simulink model "FDIA_TRAINING_39_1"  (R2021a)
settings: Solver=ode23tb  StartTime=0.0  StopTime=27  MaxStep=1/60  RelTol=1e-2  AbsTol=1e-1  EnableMultiTasking=on
PreLoadFcn:
  | NE39bus_data;
  | PSSMODEL=1;
  | LPSS=0;
  | WAPSS=0;
  | WAPSS2=0;
undefined symbols (not defined in the file): AVR_Data, D1, Delta, line, mac_con, MB, Ns, p0, Pn, s
libraries: spsThreePhaseVIMeasurementLib x40, spsThreePhasePISectionLineLib x34, simulink x20, spsGenericPowerSystemStabilizerLib x20, spsThreePhaseTransformerTwoWindingsLib x12, spsSynchronousMachinepuStandardLib x10, spsExcitationSystemLib x10, spsMultiBandPowerSystemStabilizerLib x10, spsSteamTurbineandGovernorLib x10, slpidlib x10, spsLoadFlowBusLib x9, spsThreePhaseDynamicLoadLib x9
(part 1 of 4)
settings Model: Creator=Innocent  LastModifiedBy=suman
settings SolverCC: AutoScaleAbsTol=off  AlgebraicLoopSolver=TrustRegion
settings DataIOCC: SaveFormat=Array  SignalLoggingSaveFormat=ModelDataLogs  SaveOutput=off  SaveTime=off  ReturnWorkspaceOutputs=off
settings OptimizationCC: BlockReduction=off  BooleanDataType=off  ExpressionDepthLimit=2147483647  InitFltsAndDblsToZero=on  LifeSpan=inf
settings DebuggingCC: SaveWithParameterizedLinksMsg=none  UnderspecifiedInitializationDetection=Classic  MergeDetectMultiDrivingBlocksExec=none  SignalResolutionControl=TryResolveAllWithWarning  SolverPrmCheckMsg=warning  MultiTaskDSMMsg=warning  MultiTaskCondExecSysMsg=none  FcnCallInpInsideContextMsg=warning  UnconnectedInputMsg=none  UnconnectedOutputMsg=none  UnconnectedLineMsg=none  StateNameClashWarn=warning  StrictBusMsg=ErrorOnBusTreatedAsVector  SFUnexpectedBacktrackingDiag=warning  SFNoUnconditionalDefaultTransitionDiag=warning  SFExecutionAtInitializationDiag=none  SFMachineParentedDataDiag=warning  ArithmeticOperatorsInVariantConditions=warning
settings HardwareCC: ProdBitPerPointer=32  ProdBitPerSizeT=32  ProdBitPerPtrDiffT=32  ProdLargestAtomicFloat=None  ProdIntDivRoundTo=Undefined  ProdEndianess=Unspecified  ProdWordSize=32  ProdHWDeviceType=32-bit Generic
settings ModelReferenceCC: PropagateSignalLabelsOutOfModel=off
settings SFSimCC: SimUseLocalCustomCode=off  CustomCodeUndefinedFunction=UseInterfaceOnly
settings RTWCC: RTWUseLocalCustomCode=off
settings CodeAppCC: StateflowObjectComments=on
settings GRTTargetCC: TargetFcnLib=ansi_tfl_tmw.mat  TargetLangStandard=C89/C90 (ANSI)  CombineOutputUpdateFcns=off  GRTInterface=on
settings ConfigComp: CovMetricSettings=dw  CovSaveCumulativeToWorkspaceVar=on  CovSaveSingleToWorkspaceVar=on  CovExternalEMLEnable=off
settings SimscapeCC: SimscapeNormalizeSystem=off

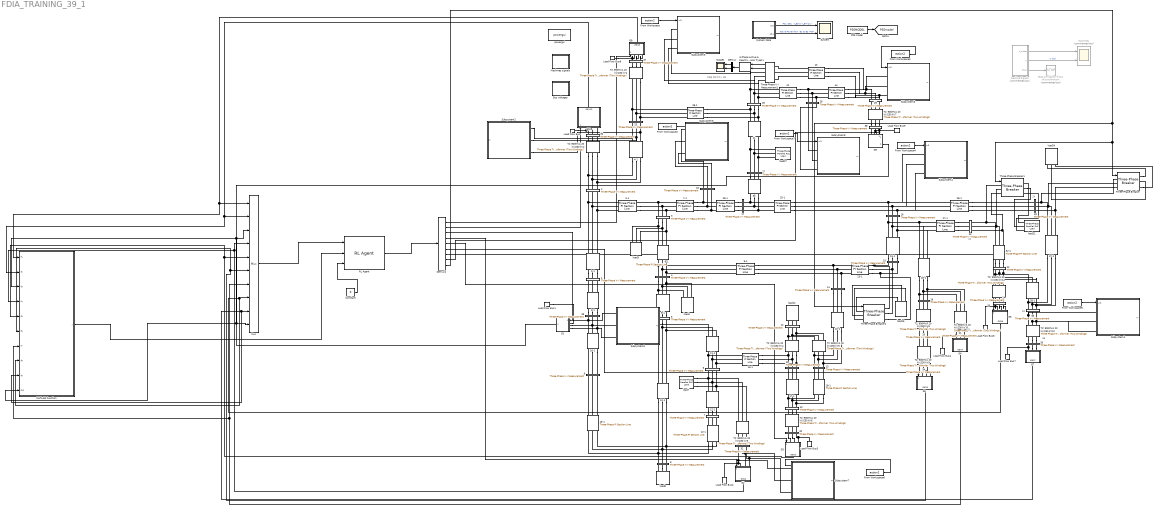
== system FDIA_TRAINING_39_1 ==
  note: 35
  note: 33
  note: 21
  note: 24
  note: 36
  note: P&Q 29 ==> 26
  note: 23
  " 30" : spsThreePhasePISectionLineLib/Three-Phase PI Section Line  LConnTagsString=a|b|c  RConnTagsString=A|B|C  Length=1  Frequency=50  Resistances="[line(30,3)  3*line(30,3)]"  Inductances="[line(30,4)  3*line(30,4)]"  Capacitances="[line(30,5)  line(30,5)/3]"
  1 : spsThreePhaseVIMeasurementLib/Three-Phase V-I Measurement  VoltageMeasurement=phase-to-phase  SetLabelV=on  LabelV=Vabc_1  Vpu=off  VpuLL=on  CurrentMeasurement=no  SetLabelI=on  LabelI=Iabc_B2  Ipu=off  Pbase=100e6  Vbase=Bus(1,2)*1e3  OutputType=Complex  PhasorSimulation=on  PSBequivalent=0
  1-1 : spsThreePhasePISectionLineLib/Three-Phase PI Section Line  LConnTagsString=a|b|c  RConnTagsString=A|B|C  Length=1  Frequency=50  Resistances="[line(1,3)  3*line(1,3)]"  Inductances="[line(1,4)  3*line(1,4)]"  Capacitances="[line(1,5)  line(1,5)/3]"
  10 : spsThreePhaseVIMeasurementLib/Three-Phase V-I Measurement  VoltageMeasurement=phase-to-phase  SetLabelV=on  LabelV=Vabc_10  Vpu=off  VpuLL=on  CurrentMeasurement=no  SetLabelI=on  LabelI=Iabc_B2  Ipu=off  Pbase=100e6  Vbase=Bus(10,2)*1e3  OutputType=Complex  PhasorSimulation=on  PSBequivalent=0
  10-1 : spsThreePhasePISectionLineLib/Three-Phase PI Section Line  LConnTagsString=a|b|c  RConnTagsString=A|B|C  Length=1  Frequency=50  Resistances="[line(10,3)  3*line(10,3)]"  Inductances="[line(10,4)  3*line(10,4)]"  Capacitances="[line(10,5)  line(10,5)/3]"
  11 : spsThreePhaseVIMeasurementLib/Three-Phase V-I Measurement  VoltageMeasurement=phase-to-phase  SetLabelV=on  LabelV=Vabc_11  Vpu=off  VpuLL=on  CurrentMeasurement=no  SetLabelI=on  LabelI=Iabc_B2  Ipu=off  Pbase=100e6  Vbase=Bus(11,2)*1e3  OutputType=Complex  PhasorSimulation=on  PSBequivalent=0
  11-1 : spsThreePhasePISectionLineLib/Three-Phase PI Section Line  LConnTagsString=a|b|c  RConnTagsString=A|B|C  Length=1  Frequency=50  Resistances="[line(11,3)  3*line(11,3)]"  Inductances="[line(11,4)  3*line(11,4)]"  Capacitances="[line(11,5)   line(11,5)/3]"
  12 : spsThreePhaseVIMeasurementLib/Three-Phase V-I Measurement  VoltageMeasurement=phase-to-phase  SetLabelV=on  LabelV=Vabc_12  Vpu=off  VpuLL=on  CurrentMeasurement=no  SetLabelI=on  LabelI=Iabc_B2  Ipu=off  Pbase=100e6  Vbase=Bus(12,2)*1e3  OutputType=Complex  PhasorSimulation=on  PSBequivalent=0
  12-1 : spsThreePhasePISectionLineLib/Three-Phase PI Section Line  LConnTagsString=a|b|c  RConnTagsString=A|B|C  Length=1  Frequency=50  Resistances="[line(12,3)  3*line(12,3)]"  Inductances="[line(12,4)  3*line(12,4)]"  Capacitances="[line(12,5)   line(12,5)/3]"
  13 : spsThreePhaseVIMeasurementLib/Three-Phase V-I Measurement  VoltageMeasurement=phase-to-phase  SetLabelV=on  LabelV=Vabc_13  Vpu=off  VpuLL=on  CurrentMeasurement=no  SetLabelI=on  LabelI=Iabc_B2  Ipu=off  Pbase=100e6  Vbase=Bus(13,2)*1e3  OutputType=Complex  PhasorSimulation=on  PSBequivalent=0
  13-1 : spsThreePhasePISectionLineLib/Three-Phase PI Section Line  LConnTagsString=a|b|c  RConnTagsString=A|B|C  Length=1  Frequency=50  Resistances=[line(13,3) 3*line(13,3)]  Inductances="[line(13,4)  3*line(13,4)]"  Capacitances="[line(13,5)  line(13,5)/3]"
  14 : spsThreePhaseVIMeasurementLib/Three-Phase V-I Measurement  VoltageMeasurement=phase-to-phase  SetLabelV=on  LabelV=Vabc_14  Vpu=off  VpuLL=on  CurrentMeasurement=no  SetLabelI=on  LabelI=Iabc_B2  Ipu=off  Pbase=100e6  Vbase=Bus(14,2)*1e3  OutputType=Complex  PhasorSimulation=on  PSBequivalent=0
  14-1 : spsThreePhasePISectionLineLib/Three-Phase PI Section Line  LConnTagsString=a|b|c  RConnTagsString=A|B|C  Length=1  Frequency=50  Resistances=[ line(14,3) 3*line(14,3)]  Inductances="[ line(14,4)  3*line(14,4)]"  Capacitances="[line(14,5)   line(14,5)/3]"
  15 : spsThreePhaseVIMeasurementLib/Three-Phase V-I Measurement  VoltageMeasurement=phase-to-phase  SetLabelV=on  LabelV=Vabc_15  Vpu=off  VpuLL=on  CurrentMeasurement=no  SetLabelI=on  LabelI=Iabc_B2  Ipu=off  Pbase=100e6  Vbase=Bus(15,2)*1e3  OutputType=Complex  PhasorSimulation=on  PSBequivalent=0
  15-1 : spsThreePhasePISectionLineLib/Three-Phase PI Section Line  LConnTagsString=a|b|c  RConnTagsString=A|B|C  Length=1  Frequency=50  Resistances="[line(15,3)  3*line(15,3)]"  Inductances="[line(15,4)  3*line(15,4)]"  Capacitances="[line(15,5)   line(15,5)/5]"
  16 : spsThreePhaseVIMeasurementLib/Three-Phase V-I Measurement  VoltageMeasurement=phase-to-phase  SetLabelV=on  LabelV=Vabc_16  Vpu=off  VpuLL=on  CurrentMeasurement=no  SetLabelI=on  LabelI=Iabc_B2  Ipu=off  Pbase=100e6  Vbase=Bus(16,2)*1e3  OutputType=Complex  PhasorSimulation=on  PSBequivalent=0
  16-1 : spsThreePhasePISectionLineLib/Three-Phase PI Section Line  LConnTagsString=a|b|c  RConnTagsString=A|B|C  Length=1  Frequency=50  Resistances="[line(8,3)  3*line(8,3)]"  Inductances="[line(8,4)  3*line(8,4)]"  Capacitances="[line(8,5)   line(8,5)/3]"
  17 : spsThreePhaseVIMeasurementLib/Three-Phase V-I Measurement  VoltageMeasurement=phase-to-phase  SetLabelV=on  LabelV=Vabc_17  Vpu=off  VpuLL=on  CurrentMeasurement=no  SetLabelI=on  LabelI=Iabc_B2  Ipu=off  Pbase=100e6  Vbase=Bus(17,2)*1e3  OutputType=Complex  PhasorSimulation=on  PSBequivalent=0
  17-1 : spsThreePhasePISectionLineLib/Three-Phase PI Section Line  LConnTagsString=a|b|c  RConnTagsString=A|B|C  Length=1  Frequency=50  Resistances="[line(17,3)  3*line(17,3)]"  Inductances="[line(17,4)  3*line(17,4)]"  Capacitances="[line(17,5)   line(17,5)/3]"
  18 : spsThreePhaseVIMeasurementLib/Three-Phase V-I Measurement  VoltageMeasurement=phase-to-phase  SetLabelV=on  LabelV=Vabc_18  Vpu=off  VpuLL=on  CurrentMeasurement=no  SetLabelI=on  LabelI=Iabc_B2  Ipu=off  Pbase=100e6  Vbase=Bus(18,2)*1e3  OutputType=Complex  PhasorSimulation=on  PSBequivalent=0
  18-1 : spsThreePhasePISectionLineLib/Three-Phase PI Section Line  LConnTagsString=a|b|c  RConnTagsString=A|B|C  Length=1  Frequency=50  Resistances="[line(18,3)  3*line(18,3)]"  Inductances="[line(18,4)  3*line(18,4)]"  Capacitances="[line(18,5)   line(18,5)/3]"
  19 : spsThreePhaseVIMeasurementLib/Three-Phase V-I Measurement  VoltageMeasurement=phase-to-phase  SetLabelV=on  LabelV=Vabc_19  Vpu=off  VpuLL=on  CurrentMeasurement=no  SetLabelI=on  LabelI=Iabc_B2  Ipu=off  Pbase=100e6  Vbase=Bus(19,2)*1e3  OutputType=Complex  PhasorSimulation=on  PSBequivalent=0
  2 : spsThreePhaseVIMeasurementLib/Three-Phase V-I Measurement  VoltageMeasurement=phase-to-phase  SetLabelV=on  LabelV=Vabc_2  Vpu=off  VpuLL=on  CurrentMeasurement=no  SetLabelI=on  LabelI=Iabc_B2  Ipu=off  Pbase=100e6  Vbase=Bus(2,2)*1e3  OutputType=Complex  PhasorSimulation=on  PSBequivalent=0
  2-1 : spsThreePhasePISectionLineLib/Three-Phase PI Section Line  LConnTagsString=a|b|c  RConnTagsString=A|B|C  Length=1  Frequency=50  Resistances="[line(2,3)  3*line(2,3)]"  Inductances="[line(2,4)  3*line(2,4)]"  Capacitances="[line(2,5)   line(2,5)/3]"
  20 : spsThreePhaseVIMeasurementLib/Three-Phase V-I Measurement  VoltageMeasurement=phase-to-phase  SetLabelV=on  LabelV=Vabc_20  Vpu=off  VpuLL=on  CurrentMeasurement=no  SetLabelI=on  LabelI=Iabc_B2  Ipu=off  Pbase=100e6  Vbase=Bus(20,2)*1e3  OutputType=Complex  PhasorSimulation=on  PSBequivalent=0
  21 : spsThreePhaseVIMeasurementLib/Three-Phase V-I Measurement  VoltageMeasurement=phase-to-phase  SetLabelV=on  LabelV=Vabc_33  Vpu=off  VpuLL=on  CurrentMeasurement=no  SetLabelI=on  LabelI=Iabc_B2  Ipu=off  Pbase=100e6  Vbase=Bus(33,2)*1e3  OutputType=Complex  PhasorSimulation=on  PSBequivalent=0
  22 : spsThreePhaseVIMeasurementLib/Three-Phase V-I Measurement  VoltageMeasurement=phase-to-phase  SetLabelV=on  LabelV=Vabc_22  Vpu=off  VpuLL=on  CurrentMeasurement=no  SetLabelI=on  LabelI=Iabc_B2  Ipu=off  Pbase=100e6  Vbase=Bus(22,2)*1e3  OutputType=Complex  PhasorSimulation=on  PSBequivalent=0
  22-1 : spsThreePhasePISectionLineLib/Three-Phase PI Section Line  LConnTagsString=a|b|c  RConnTagsString=A|B|C  Length=1  Frequency=50  Resistances="[line(22,3)  3*line(22,3)]"  Inductances="[line(22,4)  3*line(22,4)]"  Capacitances="[line(22,5)   line(22,5)/3]"
  23 : spsThreePhaseVIMeasurementLib/Three-Phase V-I Measurement  VoltageMeasurement=phase-to-phase  SetLabelV=on  LabelV=Vabc_21  Vpu=off  VpuLL=on  CurrentMeasurement=no  SetLabelI=on  LabelI=Iabc_B2  Ipu=off  Pbase=100e6  Vbase=Bus(21,2)*1e3  OutputType=Complex  PhasorSimulation=on  PSBequivalent=0
  23-1 : spsThreePhasePISectionLineLib/Three-Phase PI Section Line  LConnTagsString=a|b|c  RConnTagsString=A|B|C  Length=1  Frequency=50  Resistances="[line(23,3)  3*line(23,3)]"  Inductances="[line(23,4)  3*line(23,4)]"  Capacitances="[line(23,5)   line(23,5)/3]"
  24 : spsThreePhaseVIMeasurementLib/Three-Phase V-I Measurement  VoltageMeasurement=phase-to-phase  SetLabelV=on  LabelV=Vabc_35  Vpu=off  VpuLL=on  CurrentMeasurement=no  SetLabelI=on  LabelI=Iabc_B2  Ipu=off  Pbase=100e6  Vbase=Bus(35,2)*1e3  OutputType=Complex  PhasorSimulation=on  PSBequivalent=0
  24-1 : spsThreePhasePISectionLineLib/Three-Phase PI Section Line  LConnTagsString=a|b|c  RConnTagsString=A|B|C  Length=1  Frequency=50  Resistances="[line(24,3)  3*line(24,3)]"  Inductances="[line(24,4)  3*line(24,4)]"  Capacitances="[line(24,5)   line(24,5)/3]"
  25 : spsThreePhaseVIMeasurementLib/Three-Phase V-I Measurement  VoltageMeasurement=phase-to-phase  SetLabelV=on  LabelV=Vabc_25  Vpu=off  VpuLL=on  CurrentMeasurement=no  SetLabelI=on  LabelI=Iabc_B2  Ipu=off  Pbase=100e6  Vbase=Bus(25,2)*1e3  OutputType=Complex  PhasorSimulation=on  PSBequivalent=0
  25-1 : spsThreePhasePISectionLineLib/Three-Phase PI Section Line  LConnTagsString=a|b|c  RConnTagsString=A|B|C  Length=1  Frequency=50  Resistances="[ line(25,3)  3*line(25,3)]"  Inductances="[ line(25,4)  3*line(25,4)]"  Capacitances="[line(25,5)  line(25,5)/3]"
  26 : spsThreePhaseVIMeasurementLib/Three-Phase V-I Measurement  VoltageMeasurement=phase-to-phase  SetLabelV=on  LabelV=Vabc_26  Vpu=off  VpuLL=on  CurrentMeasurement=no  SetLabelI=on  LabelI=Iabc_B2  Ipu=off  Pbase=100e6  Vbase=Bus(26,2)*1e3  OutputType=Complex  PhasorSimulation=on  PSBequivalent=0
  26-1 : spsThreePhasePISectionLineLib/Three-Phase PI Section Line  LConnTagsString=a|b|c  RConnTagsString=A|B|C  Length=1  Frequency=50  Resistances="[line(26,3)   3*line(26,3)]"  Inductances="[line(26,4)  3*line(26,4)]"  Capacitances="[line(26,5)   line(26,5)/3]"
  27 : spsThreePhaseVIMeasurementLib/Three-Phase V-I Measurement  VoltageMeasurement=phase-to-phase  SetLabelV=on  LabelV=Vabc_27  Vpu=off  VpuLL=on  CurrentMeasurement=no  SetLabelI=on  LabelI=Iabc_B2  Ipu=off  Pbase=100e6  Vbase=Bus(27,2)*1e3  OutputType=Complex  PhasorSimulation=on  PSBequivalent=0
  27-1 : spsThreePhasePISectionLineLib/Three-Phase PI Section Line  LConnTagsString=a|b|c  RConnTagsString=A|B|C  Length=1  Frequency=50  Resistances="[line(27,3)  3*line(27,3)]"  Inductances="[line(27,4)  3*line(27,4)]"  Capacitances="[line(27,5)   line(27,5)/3]"
  28 : spsThreePhaseVIMeasurementLib/Three-Phase V-I Measurement  VoltageMeasurement=phase-to-phase  SetLabelV=on  LabelV=Vabc_28  Vpu=off  VpuLL=on  CurrentMeasurement=no  SetLabelI=on  LabelI=Iabc_B2  Ipu=off  Pbase=100e6  Vbase=Bus(28,2)*1e3  OutputType=Complex  PhasorSimulation=on  PSBequivalent=0
  28-1 : spsThreePhasePISectionLineLib/Three-Phase PI Section Line  LConnTagsString=a|b|c  RConnTagsString=A|B|C  Length=1  Frequency=50  Resistances=[line(28,3) 3*line(28,3) ]  Inductances="[line(28,4)  3*line(28,4)]"  Capacitances="[line(28,5)   line(28,5)/3]"
  29 : spsThreePhaseVIMeasurementLib/Three-Phase V-I Measurement  VoltageMeasurement=phase-to-phase  SetLabelV=on  LabelV=Vabc_29  Vpu=off  VpuLL=on  CurrentMeasurement=no  SetLabelI=on  LabelI=Iabc_B2  Ipu=off  Pbase=100e6  Vbase=Bus(29,2)*1e3  OutputType=Complex  PhasorSimulation=on  PSBequivalent=0
  29-1 : spsThreePhasePISectionLineLib/Three-Phase PI Section Line  LConnTagsString=a|b|c  RConnTagsString=A|B|C  Length=1  Frequency=50  Resistances=[ line(29,3) 3*line(29,3)]  Inductances="[ line(29,4)  3*line(29,4)]"  Capacitances="[line(29,5)    line(29,5)/3]"
  3 : spsThreePhaseVIMeasurementLib/Three-Phase V-I Measurement  VoltageMeasurement=phase-to-phase  SetLabelV=on  LabelV=Vabc_B3  Vpu=off  VpuLL=on  CurrentMeasurement=yes  SetLabelI=on  LabelI=Iabc_B3  Ipu=off  Pbase=100e6  Vbase=Bus(3,2)*1e3  OutputType=Complex  PhasorSimulation=on  PSBequivalent=0
  3-1 : spsThreePhasePISectionLineLib/Three-Phase PI Section Line  LConnTagsString=a|b|c  RConnTagsString=A|B|C  Length=1  Frequency=50  Resistances=[line(3,3) 3*line(3,3)]  Inductances="[line(3,4)  3*line(3,4)]"  Capacitances="[line(3,5)   line(3,5)/3]"
  3-Phase Active & Reactive Power (Phasor Type)1 : powerlib_extras/Phasor Library/3-Phase Active & Reactive Power (Phasor Type)
      settings: SourceProductBaseCode=PS
  30 : spsThreePhaseVIMeasurementLib/Three-Phase V-I Measurement  VoltageMeasurement=phase-to-phase  SetLabelV=on  LabelV=Vabc_30  Vpu=off  VpuLL=on  CurrentMeasurement=no  SetLabelI=on  LabelI=Iabc_B2  Ipu=off  Pbase=100e6  Vbase=Bus(30,2)*1e3  OutputType=Complex  PhasorSimulation=on  PSBequivalent=0
  31 : spsThreePhaseVIMeasurementLib/Three-Phase V-I Measurement  VoltageMeasurement=phase-to-phase  SetLabelV=on  LabelV=Vabc_31  Vpu=off  VpuLL=on  CurrentMeasurement=no  SetLabelI=on  LabelI=Iabc_B2  Ipu=off  Pbase=100e6  Vbase=Bus(31,2)*1e3  OutputType=Complex  PhasorSimulation=on  PSBequivalent=0
  32 : spsThreePhaseVIMeasurementLib/Three-Phase V-I Measurement  VoltageMeasurement=phase-to-phase  SetLabelV=on  LabelV=Vabc_32  Vpu=off  VpuLL=on  CurrentMeasurement=no  SetLabelI=on  LabelI=Iabc_B2  Ipu=off  Pbase=100e6  Vbase=Bus(32,2)*1e3  OutputType=Complex  PhasorSimulation=on  PSBequivalent=0
  33 : spsThreePhaseVIMeasurementLib/Three-Phase V-I Measurement  VoltageMeasurement=phase-to-phase  SetLabelV=on  LabelV=Vabc_24  Vpu=off  VpuLL=on  CurrentMeasurement=no  SetLabelI=on  LabelI=Iabc_B2  Ipu=off  Pbase=100e6  Vbase=Bus(24,2)*1e3  OutputType=Complex  PhasorSimulation=on  PSBequivalent=0
  34 : spsThreePhaseVIMeasurementLib/Three-Phase V-I Measurement  VoltageMeasurement=phase-to-phase  SetLabelV=on  LabelV=Vabc_34  Vpu=off  VpuLL=on  CurrentMeasurement=no  SetLabelI=on  LabelI=Iabc_B2  Ipu=off  Pbase=100e6  Vbase=Bus(34,2)*1e3  OutputType=Complex  PhasorSimulation=on  PSBequivalent=0
  34-1 : spsThreePhasePISectionLineLib/Three-Phase PI Section Line  LConnTagsString=a|b|c  RConnTagsString=A|B|C  Length=1  Frequency=50  Resistances="[line(34,3)  3*line(34,3) ]"  Inductances="[line(34,4)  3*line(34,4)]"  Capacitances="[line(34,5)   line(34,5)/3]"
  35 : spsThreePhaseVIMeasurementLib/Three-Phase V-I Measurement  VoltageMeasurement=phase-to-phase  SetLabelV=on  LabelV=Vabc_36  Vpu=off  VpuLL=on  CurrentMeasurement=no  SetLabelI=on  LabelI=Iabc_B2  Ipu=off  Pbase=100e6  Vbase=Bus(36,2)*1e3  OutputType=Complex  PhasorSimulation=on  PSBequivalent=0
  35-1 : spsThreePhasePISectionLineLib/Three-Phase PI Section Line  LConnTagsString=a|b|c  RConnTagsString=A|B|C  Length=1  Frequency=50  Resistances="[line(35,3)  3*line(35,3)]"  Inductances="[line(35,4)  3*line(35,4)]"  Capacitances="[line(35,5)   line(35,5)/3]"
  36 : spsThreePhaseVIMeasurementLib/Three-Phase V-I Measurement  VoltageMeasurement=phase-to-phase  SetLabelV=on  LabelV=Vabc_23  Vpu=off  VpuLL=on  CurrentMeasurement=no  SetLabelI=on  LabelI=Iabc_B2  Ipu=off  Pbase=100e6  Vbase=Bus(23,2)*1e3  OutputType=Complex  PhasorSimulation=on  PSBequivalent=0
  37 : spsThreePhaseVIMeasurementLib/Three-Phase V-I Measurement  VoltageMeasurement=phase-to-phase  SetLabelV=on  LabelV=Vabc_37  Vpu=off  VpuLL=on  CurrentMeasurement=no  SetLabelI=on  LabelI=Iabc_B2  Ipu=off  Pbase=100e6  Vbase=Bus(37,2)*1e3  OutputType=Complex  PhasorSimulation=on  PSBequivalent=0
  37-1 : spsThreePhasePISectionLineLib/Three-Phase PI Section Line  LConnTagsString=a|b|c  RConnTagsString=A|B|C  Length=1  Frequency=50  Resistances="[line(37,3)  3*line(37,3) ]"  Inductances="[line(37,4)  3*line(37,4)]"  Capacitances="[line(37,5)   line(37,5)/3]"
  38 : spsThreePhaseVIMeasurementLib/Three-Phase V-I Measurement  VoltageMeasurement=phase-to-phase  SetLabelV=on  LabelV=Vabc_38  Vpu=off  VpuLL=on  CurrentMeasurement=no  SetLabelI=off  LabelI=Iabc_B2  Ipu=off  Pbase=100e6  Vbase=Bus(38,2)*1e3  OutputType=Complex  PhasorSimulation=on  PSBequivalent=0
  39 : spsThreePhaseVIMeasurementLib/Three-Phase V-I Measurement  VoltageMeasurement=phase-to-phase  SetLabelV=on  LabelV=Vabc_39  Vpu=off  VpuLL=on  CurrentMeasurement=no  SetLabelI=on  LabelI=Iabc_B2  Ipu=off  Pbase=100e6  Vbase=Bus(39,2)*1e3  OutputType=Complex  PhasorSimulation=on  PSBequivalent=0
  39-1 : spsThreePhasePISectionLineLib/Three-Phase PI Section Line  LConnTagsString=a|b|c  RConnTagsString=A|B|C  Length=1  Frequency=50  Resistances=[ line(39,3) 3* line(39,3)]  Inductances="[ line(39,4)  3*line(39,4)]"  Capacitances="[line(39,5)  line(39,5)/3]"
  4 : spsThreePhaseVIMeasurementLib/Three-Phase V-I Measurement  VoltageMeasurement=phase-to-phase  SetLabelV=on  LabelV=Vabc_B4  Vpu=off  VpuLL=on  CurrentMeasurement=yes  SetLabelI=on  LabelI=Iabc_B4  Ipu=off  Pbase=100e6  Vbase=Bus(4,2)*1e3  OutputType=Complex  PhasorSimulation=on  PSBequivalent=0
  4-1 : spsThreePhasePISectionLineLib/Three-Phase PI Section Line  LConnTagsString=a|b|c  RConnTagsString=A|B|C  Length=1  Frequency=50  Resistances="[line(4,3)  3*line(4,3)]"  Inductances="[line(4,4)  3*line(4,4)]"  Capacitances="[line(4,5)   line(4,5)/3]"
  41 : spsThreePhasePISectionLineLib/Three-Phase PI Section Line  LConnTagsString=a|b|c  RConnTagsString=A|B|C  Length=1  Frequency=50  Resistances="[ line(41,3)  3*line(41,3)]"  Inductances="[ line(41,4)  3*line(41,4)]"  Capacitances="[line(41,5)    line(41,5)/3]"
  42 : spsThreePhasePISectionLineLib/Three-Phase PI Section Line  LConnTagsString=a|b|c  RConnTagsString=A|B|C  Length=1  Frequency=50  Resistances="[ line(42,3)   3*line(42,3)]"  Inductances="[ line(42,4)   3*line(42,4)]"  Capacitances="[line(42,5)    line(42,5)/3]"
  43 : spsThreePhasePISectionLineLib/Three-Phase PI Section Line  LConnTagsString=a|b|c  RConnTagsString=A|B|C  Length=1  Frequency=50  Resistances="[ line(43,3)  3* line(43,3) ]"  Inductances="[ line(43,4)   3*line(43,4)]"  Capacitances="[line(43,5)   line(43,5)/3]"
  44 : spsThreePhasePISectionLineLib/Three-Phase PI Section Line  LConnTagsString=a|b|c  RConnTagsString=A|B|C  Length=1  Frequency=50  Resistances="[ line(44,3)  3* line(44,3)]"  Inductances="[ line(44,4)  3* line(44,4)]"  Capacitances="[line(44,5)   line(44,5)/3]"
  5 : spsThreePhaseVIMeasurementLib/Three-Phase V-I Measurement  VoltageMeasurement=phase-to-phase  SetLabelV=on  LabelV=Vabc_5  Vpu=off  VpuLL=on  CurrentMeasurement=no  SetLabelI=on  LabelI=Iabc_B2  Ipu=off  Pbase=100e6  Vbase=Bus(5,2)*1e3  OutputType=Complex  PhasorSimulation=on  PSBequivalent=0
  6 : spsThreePhaseVIMeasurementLib/Three-Phase V-I Measurement  VoltageMeasurement=phase-to-phase  SetLabelV=on  LabelV=Vabc_6  Vpu=off  VpuLL=on  CurrentMeasurement=no  SetLabelI=on  LabelI=Iabc_B2  Ipu=off  Pbase=100e6  Vbase=Bus(6,2)*1e3  OutputType=Complex  PhasorSimulation=on  PSBequivalent=0
  6-1 : spsThreePhasePISectionLineLib/Three-Phase PI Section Line  LConnTagsString=a|b|c  RConnTagsString=A|B|C  Length=1  Frequency=50  Resistances="[line(6,3)    3*line(6,3) ]"  Inductances="[line(6,4)   3*line(6,4)]"  Capacitances="[line(6,5)   line(6,5)/3]"
  7 : spsThreePhaseVIMeasurementLib/Three-Phase V-I Measurement  VoltageMeasurement=phase-to-phase  SetLabelV=on  LabelV=Vabc_7  Vpu=off  VpuLL=on  CurrentMeasurement=no  SetLabelI=on  LabelI=Iabc_B2  Ipu=off  Pbase=100e6  Vbase=Bus(8,2)*1e3  OutputType=Complex  PhasorSimulation=on  PSBequivalent=0
  7-1 : spsThreePhasePISectionLineLib/Three-Phase PI Section Line  LConnTagsString=a|b|c  RConnTagsString=A|B|C  Length=1  Frequency=50  Resistances="[line(7,3)  3*line(7,3)]"  Inductances="[line(7,4)  3*line(7,4)]"  Capacitances="[line(7,5)   line(7,5)/3]"
  8 : spsThreePhaseVIMeasurementLib/Three-Phase V-I Measurement  VoltageMeasurement=phase-to-phase  SetLabelV=on  LabelV=Vabc_8  Vpu=off  VpuLL=on  CurrentMeasurement=no  SetLabelI=on  LabelI=Iabc_B2  Ipu=off  Pbase=100e6  Vbase=Bus(8,2)*1e3  OutputType=Complex  PhasorSimulation=on  PSBequivalent=0
  8-1 : spsThreePhasePISectionLineLib/Three-Phase PI Section Line  LConnTagsString=a|b|c  RConnTagsString=A|B|C  Length=1  Frequency=50  Resistances="[line(8,3)  3*line(8,3) ]"  Inductances="[line(8,4)  3*line(8,4)]"  Capacitances="[line(8,5)   line(8,5)/3]"
  9 : spsThreePhaseVIMeasurementLib/Three-Phase V-I Measurement  VoltageMeasurement=phase-to-phase  SetLabelV=on  LabelV=Vabc_9  Vpu=off  VpuLL=on  CurrentMeasurement=no  SetLabelI=on  LabelI=Iabc_B2  Ipu=off  Pbase=100e6  Vbase=Bus(9,2)*1e3  OutputType=Complex  PhasorSimulation=on  PSBequivalent=0
  9-1 : spsThreePhasePISectionLineLib/Three-Phase PI Section Line  LConnTagsString=a|b|c  RConnTagsString=A|B|C  Length=1  Frequency=50  Resistances="[ line(9,3)  3*line(9,3) ]"  Inductances="[ line(9,4)  3*line(9,4)]"  Capacitances="[line(9,5)   line(9,5)/3]"
  Bus voltages : Subsystem
  Constant : Constant  Value=0
  Demux : Demux  Outputs=2
      settings: DisplayOption=none
  Demux1 : Demux  Outputs=9
  From Workspace{,2..7} (7 alike) : FromWorkspace  VariableName=action2
  G1 : Subsystem
  G10 : Subsystem
  G2 : Subsystem
  G3 : Subsystem
  G4 : Subsystem
  G5 : Subsystem
  G6 : Subsystem
  G7 : Subsystem
  G8 : Subsystem
  G9 : Subsystem
      settings: PortSchema="{\"entries\":[{\"content\":{\"sides\":[{\"content\":{\"connectorIds\":[\"LConn1\",\"LConn2\",\"LConn3\",\"In1\"]},\"type\":\"ConnectorPlacement.EquallySpacedRectSide\",\"uuid\":\"0ca931fd-618d-409d-a3a8-1be2e3c1cf8f\"},{\"content\":{\"connectorIds\":[],\"side\":\"RIGHT\"},\"type\":\"ConnectorPlacement.EquallySpacedRectSide\",\"uuid\":\"41042dbf-c308-4e32-8c77-0486dcc0e60b\"},{\"content\":{\"connectorIds\":[],\"side\":\"TOP\"},\"type\":\"ConnectorPlacement.EquallySpacedRectSide\",\"uuid\":\"3f3fed6c-9036-4c19-8432-555009ec3b0d\"},{\"content\":{\"connectorIds\":[\"Out1\",\"Out2\"],\"side\":\"BOTTOM\"},\"type\":\"ConnectorPlacement.EquallySpacedRectSide\",\"uuid\":\"8c6465a4-2fe3-44c7-94a5-9cf039219e54\"}]},\"type\":\"ConnectorPlacement.EquallySpacedConnector\",\"uuid\":\"e4db8a85-161f-4ec5-8ef6-84198ae69e00\"}],\"packageUris\":[\"http://schema.mathworks.com/mf0/Connector/R2020b\"],\"version\":\"1.0\"}"
  Load Flow Bus : spsLoadFlowBusLib/Load Flow Bus  LConnTagsString=a  Phases=single  Connectors=on one side  ID=B30  Vbase=22e3  Vref=1.0475  Vangle=0  VLF=1.048  VLFb=1  VLFc=1  angleLF=-3.646  angleLFb=0  angleLFc=0
      settings: AttributesFormatString=%<ID>\n%<Vbase>\n%<VLF>pu\n%<angleLF>deg.  SourceProductBaseCode=PS
  Load Flow Bus1 : spsLoadFlowBusLib/Load Flow Bus  LConnTagsString=a  Phases=single  Connectors=on one side  ID=Bus39  Vbase=345e3  Vref=1.03  Vangle=0  VLF=1.03  VLFb=1  VLFc=1  angleLF=19.62  angleLFb=0  angleLFc=0
      settings: AttributesFormatString=%<ID>\n%<Vbase>V\n%<VLF>pu\n%<angleLF>deg.  SourceProductBaseCode=PS
  Load Flow Bus2 : spsLoadFlowBusLib/Load Flow Bus  LConnTagsString=a  Phases=single  Connectors=on one side  ID=Bus31  Vbase=22e3  Vref=0.9820  Vangle=0  VLF=0.982  VLFb=1  VLFc=1  angleLF=0  angleLFb=0  angleLFc=0
      settings: AttributesFormatString=%<ID>\n%<Vbase>V\n%<VLF>pu\n%<angleLF>deg.  SourceProductBaseCode=PS
  Load Flow Bus3 : spsLoadFlowBusLib/Load Flow Bus  LConnTagsString=a  Phases=single  Connectors=on one side  ID=Bus32  Vbase=22e3  Vref=0.9831  Vangle=0  VLF=0.9831  VLFb=1  VLFc=1  angleLF=2.466  angleLFb=0  angleLFc=0
      settings: AttributesFormatString=%<ID>\n%<Vbase>V\n%<VLF>pu\n%<angleLF>deg.  SourceProductBaseCode=PS
  Load Flow Bus4 : spsLoadFlowBusLib/Load Flow Bus  LConnTagsString=a  Phases=single  Connectors=on one side  ID=Bus33  Vbase=22e3  Vref=0.9972  Vangle=0  VLF=0.9972  VLFb=1  VLFc=1  angleLF=4.423  angleLFb=0  angleLFc=0
      settings: AttributesFormatString=%<ID>\n%<Vbase>V\n%<VLF>pu\n%<angleLF>deg.  SourceProductBaseCode=PS
  Load Flow Bus6 : spsLoadFlowBusLib/Load Flow Bus  LConnTagsString=a  Phases=single  Connectors=on one side  ID=Bus35  Vbase=22e3  Vref=1.0493  Vangle=0  VLF=1.049  VLFb=1  VLFc=1  angleLF=5.698  angleLFb=0  angleLFc=0
      settings: AttributesFormatString=%<ID>\n%<Vbase>V\n%<VLF>pu\n%<angleLF>deg.  SourceProductBaseCode=PS
  Load Flow Bus7 : spsLoadFlowBusLib/Load Flow Bus  LConnTagsString=a  Phases=single  Connectors=on one side  ID=Bus36  Vbase=22e3  Vref=1.0635  Vangle=0  VLF=1.063  VLFb=1  VLFc=1  angleLF=8.494  angleLFb=0  angleLFc=0
      settings: AttributesFormatString=%<ID>\n%<Vbase>V\n%<VLF>pu\n%<angleLF>deg.  SourceProductBaseCode=PS
  Load Flow Bus8 : spsLoadFlowBusLib/Load Flow Bus  LConnTagsString=a  Phases=single  Connectors=on one side  ID=Bus37  Vbase=22e3  Vref=1.0278  Vangle=0  VLF=1.028  VLFb=1  VLFc=1  angleLF=2.181  angleLFb=0  angleLFc=0
      settings: AttributesFormatString=%<ID>\n%<Vbase>V\n%<VLF>pu\n%<angleLF>deg.  SourceProductBaseCode=PS
  Load Flow Bus9 : spsLoadFlowBusLib/Load Flow Bus  LConnTagsString=a  Phases=single  Connectors=on one side  ID=Bus38  Vbase=22e3  Vref=1.0265  Vangle=0  VLF=1.027  VLFb=1  VLFc=1  angleLF=7.784  angleLFb=0  angleLFc=0
      settings: AttributesFormatString=%<ID>\n%<Vbase>V\n%<VLF>pu\n%<angleLF>deg.  SourceProductBaseCode=PS
  MATLAB Function : MATLAB Function  TreatAsAtomicUnit=on
  Machine Signals : Subsystem  Commented=on
  Machines : Scope  Commented=on  NumInputPorts=2
  Machines signals : Subsystem
  Mux : Mux  Inputs=10
  PSS model : Constant  Value=PSSMODEL
  RL Agent : rllib/RL Agent  Agent=agentFDIA_39  ExternalActionAsInput=off  ProvideCumRwd=off  TreatAsDirectFeedthrough=on
  Scope1 : Scope  NumInputPorts=2
  Stop simulation if loss of synchronism : Stop  Commented=on
  Subsystem1 : Subsystem
      mask Display: image('C:\Users\suman\Downloads\Gridsense-Line-IQ-Advanced-Distribution-Submission-Line-Monitoring-2.jpg'); % Use "Edit Image" on toolstrip to change.
  Subsystem2 : Subsystem
      mask Display: image('C:\Users\suman\Downloads\Gridsense-Line-IQ-Advanced-Distribution-Submission-Line-Monitoring-2.jpg'); % Use "Edit Image" on toolstrip to change.
  Subsystem3 : Subsystem
      mask Display: image('C:\Users\suman\Downloads\Gridsense-Line-IQ-Advanced-Distribution-Submission-Line-Monitoring-2.jpg'); % Use "Edit Image" on toolstrip to change.
  Subsystem4 : Subsystem
      mask Display: image('C:\Users\suman\Downloads\Gridsense-Line-IQ-Advanced-Distribution-Submission-Line-Monitoring-2.jpg'); % Use "Edit Image" on toolstrip to change.
  Subsystem5 : Subsystem
      mask Display: image('C:\Users\suman\Downloads\Gridsense-Line-IQ-Advanced-Distribution-Submission-Line-Monitoring-2.jpg'); % Use "Edit Image" on toolstrip to change.
  Subsystem6 : Subsystem
      mask Display: image('C:\Users\suman\Downloads\Gridsense-Line-IQ-Advanced-Distribution-Submission-Line-Monitoring-2.jpg'); % Use "Edit Image" on toolstrip to change.
  Subsystem7 : Subsystem
      mask Display: image('C:\Users\suman\Downloads\Gridsense-Line-IQ-Advanced-Distribution-Submission-Line-Monitoring-2.jpg'); % Use "Edit Image" on toolstrip to change.
  Subsystem8 : Subsystem
      mask Display: image('C:\Users\suman\Downloads\Gridsense-Line-IQ-Advanced-Distribution-Submission-Line-Monitoring-2.jpg'); % Use "Edit Image" on toolstrip to change.
  Subsystem9 : Subsystem
      mask Display: image('C:\Users\suman\Downloads\Gridsense-Line-IQ-Advanced-Distribution-Submission-Line-Monitoring-2.jpg'); % Use "Edit Image" on toolstrip to change.
  System : Scope  NumInputPorts=2
  System Data : Subsystem
  T2: 900MVA 20 kV/230 kV1 : spsThreePhaseTransformerTwoWindingsLib/Three-Phase Transformer (Two Windings)  Winding1Connection=Delta (D1)  Winding2Connection=Yg  CoreType=Three single-phase transformers  SetSaturation=off  Hysteresis=off  DataFile='hysteresis'  SetInitialFlux=off  Measurements=None  UNITS=pu  NominalPower=[ 1000e6 50 ]  Winding1="[ 22e3*1.0 0.0003*s  0]"  Winding2="[ 345e3*1.0 0.0003*s  0.0232*s]"  Rm=500  Lm=500  L0=0.5  Saturation="[ 0,0  ;  0.005,1.2  ;  1.0,1.4 ]"  InitialFluxes=[ 0.8 , -0.8 , 0.7 ]  BreakLoop=off  DiscreteSolver=Trapezoidal iterative  DataType=off  TransfoNumber=0
  T2: 900MVA 20 kV/230 kV10 : spsThreePhaseTransformerTwoWindingsLib/Three-Phase Transformer (Two Windings)  Winding1Connection=Delta (D1)  Winding2Connection=Yg  CoreType=Three single-phase transformers  SetSaturation=off  Hysteresis=off  DataFile='hysteresis'  SetInitialFlux=off  Measurements=None  UNITS=pu  NominalPower=[ 1000e6 50 ]  Winding1="[ 22e3*1.0   0.00035*s  0]"  Winding2="[ 345e3*1.0  0.00035*s  0.0142*s]"  Rm=500  Lm=500  L0=0.5  Saturation="[ 0,0  ;  0.005,1.2  ;  1.0,1.4 ]"  InitialFluxes=[ 0.8 , -0.8 , 0.7 ]  BreakLoop=off  DiscreteSolver=Trapezoidal iterative  DataType=off  TransfoNumber=0
  T2: 900MVA 20 kV/230 kV11 : spsThreePhaseTransformerTwoWindingsLib/Three-Phase Transformer (Two Windings)  Winding1Connection=Delta (D1)  Winding2Connection=Yg  CoreType=Three single-phase transformers  SetSaturation=off  Hysteresis=off  DataFile='hysteresis'  SetInitialFlux=off  Measurements=None  UNITS=pu  NominalPower=[ 1000e6 50 ]  Winding1="[ 22e3*1.0  1e-6  0]"  Winding2="[ 345e3*1.0  1e-6  0.0143*s]"  Rm=500  Lm=500  L0=0.5  Saturation="[ 0,0  ;  0.005,1.2  ;  1.0,1.4 ]"  InitialFluxes=[ 0.8 , -0.8 , 0.7 ]  BreakLoop=off  DiscreteSolver=Trapezoidal iterative  DataType=off  TransfoNumber=0
  T2: 900MVA 20 kV/230 kV12 : spsThreePhaseTransformerTwoWindingsLib/Three-Phase Transformer (Two Windings)  Winding1Connection=Delta (D1)  Winding2Connection=Yg  CoreType=Three single-phase transformers  SetSaturation=off  Hysteresis=off  DataFile='hysteresis'  SetInitialFlux=off  Measurements=None  UNITS=pu  NominalPower=[ 1000e6 50 ]  Winding1="[ 22e3    0.00025*s  0.0]"  Winding2="[ 345e3    0.00025*s  0.0272*s]"  Rm=500  Lm=500  L0=0.5  Saturation="[ 0,0  ;  0.005,1.2  ;  1.0,1.4 ]"  InitialFluxes=[ 0.8 , -0.8 , 0.7 ]  BreakLoop=off  DiscreteSolver=Trapezoidal iterative  DataType=off  TransfoNumber=0
  T2: 900MVA 20 kV/230 kV2 : spsThreePhaseTransformerTwoWindingsLib/Three-Phase Transformer (Two Windings)  Winding1Connection=Delta (D1)  Winding2Connection=Yg  CoreType=Three single-phase transformers  SetSaturation=off  Hysteresis=off  DataFile='hysteresis'  SetInitialFlux=off  Measurements=None  UNITS=pu  NominalPower=[ 1000e6 50 ]  Winding1="[ 22e3*1.0  1e-6  0]"  Winding2="[ 345e3*1.0  1e-6  0.0181*s]"  Rm=500  Lm=500  L0=0.5  Saturation="[ 0,0  ;  0.005,1.2  ;  1.0,1.4 ]"  InitialFluxes=[ 0.8 , -0.8 , 0.7 ]  BreakLoop=off  DiscreteSolver=Trapezoidal iterative  DataType=off  TransfoNumber=0
  T2: 900MVA 20 kV/230 kV3 : spsThreePhaseTransformerTwoWindingsLib/Three-Phase Transformer (Two Windings)  Winding1Connection=Delta (D1)  Winding2Connection=Yg  CoreType=Three single-phase transformers  SetSaturation=off  Hysteresis=off  DataFile='hysteresis'  SetInitialFlux=off  Measurements=None  UNITS=pu  NominalPower=[ 1000e6 50 ]  Winding1="[ 22e3*1.0 1e-6  0]"  Winding2="[ 345e3*1.0  1e-6  0.0250*s ]"  Rm=500  Lm=500  L0=0.5  Saturation="[ 0,0  ;  0.005,1.2  ;  1.0,1.4 ]"  InitialFluxes=[ 0.8 , -0.8 , 0.7 ]  BreakLoop=off  DiscreteSolver=Trapezoidal iterative  DataType=off  TransfoNumber=0
  T2: 900MVA 20 kV/230 kV4 : spsThreePhaseTransformerTwoWindingsLib/Three-Phase Transformer (Two Windings)  Winding1Connection=Y  Winding2Connection=Y  CoreType=Three single-phase transformers  SetSaturation=off  Hysteresis=off  DataFile='hysteresis'  SetInitialFlux=off  Measurements=None  UNITS=pu  NominalPower=[ 1000e6 50 ]  Winding1="[ 345e3 .0008*s  0]"  Winding2="[ 230e3*1.00  .0008*s   .0435*s]"  Rm=500  Lm=500  L0=0.5  Saturation="[ 0,0  ;  0.005,1.2  ;  1.0,1.4 ]"  InitialFluxes=[ 0.8 , -0.8 , 0.7 ]  BreakLoop=off  DiscreteSolver=Trapezoidal iterative  DataType=off  TransfoNumber=0
  T2: 900MVA 20 kV/230 kV5 : spsThreePhaseTransformerTwoWindingsLib/Three-Phase Transformer (Two Windings)  Winding1Connection=Y  Winding2Connection=Y  CoreType=Three single-phase transformers  SetSaturation=off  Hysteresis=off  DataFile='hysteresis'  SetInitialFlux=off  Measurements=None  UNITS=pu  NominalPower=[ 1000e6 50 ]  Winding1="[ 345e3 .0008*s  0]"  Winding2="[ 230e3*1.00 .0008*s  .0435*s]"  Rm=500  Lm=500  L0=0.5  Saturation="[ 0,0  ;  0.005,1.2  ;  1.0,1.4 ]"  InitialFluxes=[ 0.8 , -0.8 , 0.7 ]  BreakLoop=off  DiscreteSolver=Trapezoidal iterative  DataType=off  TransfoNumber=0
  T2: 900MVA 20 kV/230 kV6 : spsThreePhaseTransformerTwoWindingsLib/Three-Phase Transformer (Two Windings)  Winding1Connection=Delta (D1)  Winding2Connection=Yg  CoreType=Three single-phase transformers  SetSaturation=off  Hysteresis=off  DataFile='hysteresis'  SetInitialFlux=off  Measurements=None  UNITS=pu  NominalPower=[ 1000e6 50 ]  Winding1="[ 22e3*1.0 1e-6  0]"  Winding2="[ 345e3*1.0   1e-6    0.020*s*1.0 ]"  Rm=500  Lm=500  L0=0.5  Saturation="[ 0,0  ;  0.005,1.2  ;  1.0,1.4 ]"  InitialFluxes=[ 0.8 , -0.8 , 0.7 ]  BreakLoop=off  DiscreteSolver=Trapezoidal iterative  DataType=off  TransfoNumber=0
  T2: 900MVA 20 kV/230 kV7 : spsThreePhaseTransformerTwoWindingsLib/Three-Phase Transformer (Two Windings)  Winding1Connection=Delta (D1)  Winding2Connection=Yg  CoreType=Three single-phase transformers  SetSaturation=off  Hysteresis=off  DataFile='hysteresis'  SetInitialFlux=off  Measurements=None  UNITS=pu  NominalPower=[ 1000e6 50 ]  Winding1="[ 22e3*1.  0.0004*s  0]"  Winding2="[ 345e3*1.0  0.0004*s  0.0156*s]"  Rm=500  Lm=500  L0=0.5  Saturation="[ 0,0  ;  0.005,1.2  ;  1.0,1.4 ]"  InitialFluxes=[ 0.8 , -0.8 , 0.7 ]  BreakLoop=off  DiscreteSolver=Trapezoidal iterative  DataType=off  TransfoNumber=0
  T2: 900MVA 20 kV/230 kV8 : spsThreePhaseTransformerTwoWindingsLib/Three-Phase Transformer (Two Windings)  Winding1Connection=Y  Winding2Connection=Y  CoreType=Three single-phase transformers  SetSaturation=off  Hysteresis=off  DataFile='hysteresis'  SetInitialFlux=off  Measurements=None  UNITS=pu  NominalPower=[ 1000e6 50 ]  Winding1="[ 345e3*1.0  0.00035*s   0]"  Winding2="[ 345e3*1.00 0.00035*s  0.0138*s]"  Rm=500  Lm=500  L0=0.5  Saturation="[ 0,0  ;  0.005,1.2  ;  1.0,1.4 ]"  InitialFluxes=[ 0.8 , -0.8 , 0.7 ]  BreakLoop=off  DiscreteSolver=Trapezoidal iterative  DataType=off  TransfoNumber=0
  T2: 900MVA 20 kV/230 kV9 : spsThreePhaseTransformerTwoWindingsLib/Three-Phase Transformer (Two Windings)  Winding1Connection=Delta (D1)  Winding2Connection=Yg  CoreType=Three single-phase transformers  SetSaturation=off  Hysteresis=off  DataFile='hysteresis'  SetInitialFlux=off  Measurements=None  UNITS=pu  NominalPower=[ 1000e6 50 ]  Winding1="[ 22e3*1.00 0.00045*s  0]"  Winding2="[ 345e3*1  0.00045*s  0.0180*s]"  Rm=500  Lm=500  L0=0.5  Saturation="[ 0,0  ;  0.005,1.2  ;  1.0,1.4 ]"  InitialFluxes=[ 0.8 , -0.8 , 0.7 ]  BreakLoop=off  DiscreteSolver=Trapezoidal iterative  DataType=off  TransfoNumber=0
  Three-Phase V-I Measurement1 : spsThreePhaseVIMeasurementLib/Three-Phase V-I Measurement  VoltageMeasurement=phase-to-ground  SetLabelV=off  LabelV=Vabc  Vpu=off  VpuLL=off  CurrentMeasurement=yes  SetLabelI=off  LabelI=Iabc  Ipu=off  Pbase=100e6  Vbase=500e3  OutputType=Complex  PhasorSimulation=on  PSBequivalent=0
  Three-Phase Breaker : spsThreePhaseBreakerLib/Three-Phase Breaker  InitialState=open  SwitchA=on  SwitchB=on  SwitchC=on  SwitchTimes="[1/60  5/60]"  External=on  BreakerResistance=0.01  SnubberResistance=1e6  SnubberCapacitance=inf  Measurements=None
  Three-Phase Breaker1 : spsThreePhaseBreakerLib/Three-Phase Breaker  InitialState=open  SwitchA=on  SwitchB=on  SwitchC=on  SwitchTimes="[1/60  5/60]"  External=on  BreakerResistance=0.01  SnubberResistance=1e6  SnubberCapacitance=inf  Measurements=None
  Three-Phase Breaker2 : spsThreePhaseBreakerLib/Three-Phase Breaker  InitialState=open  SwitchA=on  SwitchB=on  SwitchC=on  SwitchTimes="[1/60  5/60]"  External=on  BreakerResistance=0.01  SnubberResistance=1e6  SnubberCapacitance=inf  Measurements=None
  load12 : spsThreePhaseParallelRLCLoadLib/Three-Phase Parallel RLC Load  LConnTagsString=A|B|C  Configuration=Y (grounded)  NominalVoltage=(230000)*0.939625  Vabc=[1e3 1e3 1e3]  Vabcp=[1e3 1e3 1e3]  NominalFrequency=50  UnbalancedPower=off  ActivePower=7.5e6  InductivePower=88e6  CapacitivePower=0  Pabc=[10e3 9e3 11e3]  QLabc=[100 90 110]  QCabc=[100 90 110]  Pabcp=[10e3 9e3 11e3]  QLabcp=[100 90 110]  QCabcp=[100 90 110]  Measurements=None  LoadType=constant PQ
  load15 : spsThreePhaseParallelRLCLoadLib/Three-Phase Parallel RLC Load  LConnTagsString=A|B|C  Configuration=Y (grounded)  NominalVoltage=(345000)*0.969586  Vabc=[1e3 1e3 1e3]  Vabcp=[1e3 1e3 1e3]  NominalFrequency=50  UnbalancedPower=off  ActivePower=320e6  InductivePower=153e6  CapacitivePower=0  Pabc=[10e3 9e3 11e3]  QLabc=[100 90 110]  QCabc=[100 90 110]  Pabcp=[10e3 9e3 11e3]  QLabcp=[100 90 110]  QCabcp=[100 90 110]  Measurements=None  LoadType=constant PQ
  load21 : spsThreePhaseParallelRLCLoadLib/Three-Phase Parallel RLC Load  LConnTagsString=A|B|C  Configuration=Y (grounded)  NominalVoltage=(345000)*0.995503  Vabc=[1e3 1e3 1e3]  Vabcp=[1e3 1e3 1e3]  NominalFrequency=50  UnbalancedPower=off  ActivePower=274e6  InductivePower=115e6  CapacitivePower=0  Pabc=[10e3 9e3 11e3]  QLabc=[100 90 110]  QCabc=[100 90 110]  Pabcp=[10e3 9e3 11e3]  QLabcp=[100 90 110]  QCabcp=[100 90 110]  Measurements=None  LoadType=constant PQ
  load24 : spsThreePhaseParallelRLCLoadLib/Three-Phase Parallel RLC Load  LConnTagsString=A|B|C  Configuration=Y (grounded)  NominalVoltage=(345000)*0.996934  Vabc=[1e3 1e3 1e3]  Vabcp=[1e3 1e3 1e3]  NominalFrequency=50  UnbalancedPower=off  ActivePower=308.6e6  InductivePower=0  CapacitivePower=92e6  Pabc=[10e3 9e3 11e3]  QLabc=[100 90 110]  QCabc=[100 90 110]  Pabcp=[10e3 9e3 11e3]  QLabcp=[100 90 110]  QCabcp=[100 90 110]  Measurements=None  LoadType=constant PQ
  load27 : spsThreePhaseParallelRLCLoadLib/Three-Phase Parallel RLC Load  LConnTagsString=A|B|C  Configuration=Y (grounded)  NominalVoltage=(345000)*1.00029  Vabc=[1e3 1e3 1e3]  Vabcp=[1e3 1e3 1e3]  NominalFrequency=50  UnbalancedPower=off  ActivePower=281e6  InductivePower=75.5e6  CapacitivePower=0  Pabc=[10e3 9e3 11e3]  QLabc=[100 90 110]  QCabc=[100 90 110]  Pabcp=[10e3 9e3 11e3]  QLabcp=[100 90 110]  QCabcp=[100 90 110]  Measurements=None  LoadType=constant PQ
  load3 : spsThreePhaseParallelRLCLoadLib/Three-Phase Parallel RLC Load  LConnTagsString=A|B|C  Configuration=Y (grounded)  NominalVoltage=(345000)*0.992094  Vabc=[1e3 1e3 1e3]  Vabcp=[1e3 1e3 1e3]  NominalFrequency=50  UnbalancedPower=off  ActivePower=322e6  InductivePower=2.4e6  CapacitivePower=0  Pabc=[10e3 9e3 11e3]  QLabc=[100 90 110]  QCabc=[100 90 110]  Pabcp=[10e3 9e3 11e3]  QLabcp=[100 90 110]  QCabcp=[100 90 110]  Measurements=None  LoadType=constant PQ
  load4 : spsThreePhaseParallelRLCLoadLib/Three-Phase Parallel RLC Load  LConnTagsString=A|B|C  Configuration=Y (grounded)  NominalVoltage=(345000)*0.95637  Vabc=[1e3 1e3 1e3]  Vabcp=[1e3 1e3 1e3]  NominalFrequency=50  UnbalancedPower=off  ActivePower=500e6  InductivePower=184e6  CapacitivePower=0  Pabc=[10e3 9e3 11e3]  QLabc=[100 90 110]  QCabc=[100 90 110]  Pabcp=[10e3 9e3 11e3]  QLabcp=[100 90 110]  QCabcp=[100 90 110]  Measurements=None  LoadType=constant PQ
  load7 : spsThreePhaseParallelRLCLoadLib/Three-Phase Parallel RLC Load  LConnTagsString=A|B|C  Configuration=Y (grounded)  NominalVoltage=(345000)*0.956463  Vabc=[1e3 1e3 1e3]  Vabcp=[1e3 1e3 1e3]  NominalFrequency=50  UnbalancedPower=off  ActivePower=233e6  InductivePower=84e6  CapacitivePower=0  Pabc=[10e3 9e3 11e3]  QLabc=[100 90 110]  QCabc=[100 90 110]  Pabcp=[10e3 9e3 11e3]  QLabcp=[100 90 110]  QCabcp=[100 90 110]  Measurements=None  LoadType=constant PQ
  load8 : spsThreePhaseParallelRLCLoadLib/Three-Phase Parallel RLC Load  LConnTagsString=A|B|C  Configuration=Y (grounded)  NominalVoltage=(345000)*0.954036  Vabc=[1e3 1e3 1e3]  Vabcp=[1e3 1e3 1e3]  NominalFrequency=50  UnbalancedPower=off  ActivePower=522e6  InductivePower=176e6  CapacitivePower=0  Pabc=[10e3 9e3 11e3]  QLabc=[100 90 110]  QCabc=[100 90 110]  Pabcp=[10e3 9e3 11e3]  QLabcp=[100 90 110]  QCabcp=[100 90 110]  Measurements=None  LoadType=constant PQ
  powergui : spspowerguiLib/powergui  Priority=2  SimulationMode=Discrete phasor  SampleTime=1e-3  frequency=60  Iterations=50  frequencyindice=50  Pbase=100e6  ErrMax=0.0001  UnitsV=kV  UnitsW=MW  buscounter=0  FunctionMessages=off  echomessages=off  EnableUseOfTLC=off  CurrentSourceSwitches=off  DisableSnubberDevices=off  DisableRonSwitches=off  DisableVfSwitches=off  DisplayEquations=off  AutomaticDiscreteSolvers=off  SolverType=Tustin  Interpol=off  ExternalGateDelay=off  methode=off  Ts=0  x0status=blocks  SPID=off  SwTol=0  HookPort=off  NonlinearTolerance=1e-4  nMaxIteration=100  ContinueOnMaxIteration=off  RestoreLinks=warning  ResistiveCurrentMeasurement=off  Frange=logspace(0,3,50)  Ylog=off  Xlog=off  ShowGrid=off  save=off  variable=ZData  structure=0  ZoomFFT=on  StartTime=0.0  cycles=1  DisplayStyle=1  fundamental=60  FreqAxis=off  MaxFrequency=1000  frequencyindicesteady=1  RmsSteady=1  display=off
  tag scope: PSSmodel=global
  wires:
  Demux/1 -> Scope1/1
  Demux/2 -> Scope1/2
  3-Phase Active & Reactive Power (Phasor Type)1/1 -> Demux/1
  Three-Phase V-I Measurement1/1 -> 3-Phase Active & Reactive Power (Phasor Type)1/1
  Three-Phase V-I Measurement1/2 -> 3-Phase Active & Reactive Power (Phasor Type)1/2
  PSS model/1 -> [PSSmodel]
  System Data/1(Vps) -> System/1  "Pos. Seq.  V_B3 & V_B4 (pu)"
  System Data/2(p34) -> System/2  "Active Power from  B1 to B2 (MW)"
  From Workspace5/1 -> Subsystem1/1(In3)
  From Workspace3/1 -> Subsystem3/1(In3)
  From Workspace4/1 -> Subsystem4/1(In3)
  From Workspace/1 -> Subsystem5/1(In3)
  Machine Signals/2(w) -> Machines/2  "w (pu)"
  Machine Signals/1(d_theta) -> Machines/1
  Machine Signals/3(Stop) -> Stop simulation if loss of synchronism/1
  From Workspace2/1 -> ?
  From Workspace6/1 -> ?
  From Workspace7/1 -> Subsystem8/1(In3)
  Demux1/9 -> Three-Phase Breaker/1, Three-Phase Breaker1/1, Three-Phase Breaker2/1
  G8/1(GEN8) -> MATLAB Function/1(f1), Mux/1
  G10/1("GEN10 ") -> MATLAB Function/2(f2), Mux/2
  G1/1(GEN1) -> Mux/3, MATLAB Function/3(f3)
  G2/1(GEN2) -> MATLAB Function/4(f4), Mux/4
  G3/1(GEN3) -> MATLAB Function/5(f5), Mux/5
  G5/1(GEN5) -> MATLAB Function/6(f6), Mux/6
  G4/1(GEN4) -> Mux/7, MATLAB Function/7(f7)
  G6/1(GEN6) -> MATLAB Function/8(f8), Mux/8
  G7/1(GEN7) -> MATLAB Function/9(f9), Mux/9
  Mux/1 -> RL Agent/1
  RL Agent/1 -> Demux1/1
  Demux1/1 -> G8/1(DFG8)
  Demux1/2 -> G10/1(DFG10)
  Demux1/3 -> G1/1(DFG1)
  Demux1/4 -> G2/1(DFG2)
  Demux1/5 -> G3/1(DFG3)
  Demux1/6 -> G5/1(DFG5)
  Demux1/7 -> G6/1(DFG6)
  Demux1/8 -> G9/1(DFG9)
  Constant/1 -> RL Agent/3
  MATLAB Function/1(y) -> RL Agent/2
  G9/2(GEN9) -> Mux/10, MATLAB Function/10(f10)
  connections:
  16-1/LConn2 -- Subsystem9/LConn2 -- 39/RConn2 -- G1/LConn2
  16-1/LConn3 -- Subsystem9/LConn3 -- G1/LConn3 -- 39/RConn3
  39/RConn1 -- Subsystem9/LConn1 -- 16-1/LConn1 -- Load Flow Bus1/LConn1 -- G1/LConn1
  10-1/RConn1 -- 8/LConn1 -- 14-1/RConn1 -- 15-1/RConn1
  10-1/RConn2 -- 8/LConn2 -- 15-1/RConn2 -- 14-1/RConn2
  10-1/RConn3 -- 8/LConn3 -- 15-1/RConn3 -- 14-1/RConn3
  9/LConn1 -- 16-1/RConn1
  2-1/LConn3 -- 1/RConn3
  2-1/LConn2 -- 1/RConn2
  2-1/RConn1 -- 39/LConn1
  2-1/RConn2 -- 39/LConn2
  2-1/RConn3 -- 39/LConn3
  2-1/LConn1 -- 1/RConn1
  16-1/RConn3 -- 9/LConn3
  16-1/RConn2 -- 9/LConn2
  15-1/LConn1 -- 9/RConn1
  15-1/LConn3 -- 9/RConn3
  15-1/LConn2 -- 9/RConn2
  32/RConn3 -- Load Flow Bus3/LConn1 -- G3/LConn3
  32/RConn2 -- G3/LConn2
  32/RConn1 -- G3/LConn1
  17-1/RConn1 -- 18-1/RConn1 -- 10/LConn1
  17-1/RConn2 -- 18-1/RConn2 -- 10/LConn2
  17-1/RConn3 -- 18-1/RConn3 -- 10/LConn3
  G2/LConn2 -- 31/RConn2 -- Subsystem7/LConn2
  G2/LConn3 -- 31/RConn3 -- Subsystem7/LConn3
  T2: 900MVA 20 kV/230 kV4/LConn1 -- 11/LConn1 -- 13-1/RConn1
  T2: 900MVA 20 kV/230 kV4/LConn2 -- 11/LConn2 -- 13-1/RConn2
  13/LConn1 -- 22-1/RConn1 -- T2: 900MVA 20 kV/230 kV5/LConn1
  13/LConn2 -- 22-1/RConn2 -- T2: 900MVA 20 kV/230 kV5/LConn2
  22-1/RConn3 -- T2: 900MVA 20 kV/230 kV5/LConn3 -- 13/LConn3
  12-1/LConn1 -- T2: 900MVA 20 kV/230 kV3/RConn1 -- load7/LConn1 -- 6/RConn1
  12-1/LConn2 -- T2: 900MVA 20 kV/230 kV3/RConn2 -- load7/LConn2 -- 6/RConn2
  32/LConn1 -- T2: 900MVA 20 kV/230 kV6/LConn1
  10/RConn2 -- T2: 900MVA 20 kV/230 kV6/RConn2
  18-1/LConn2 -- 13/RConn2
  T2: 900MVA 20 kV/230 kV6/RConn3 -- 10/RConn3
  T2: 900MVA 20 kV/230 kV6/RConn1 -- 10/RConn1
  32/LConn2 -- T2: 900MVA 20 kV/230 kV6/LConn2
  32/LConn3 -- T2: 900MVA 20 kV/230 kV6/LConn3
  18-1/LConn1 -- 13/RConn1
  18-1/LConn3 -- 13/RConn3
  17-1/LConn3 -- 11/RConn3
  11-1/RConn2 -- 6/LConn2 -- 13-1/LConn2
  17-1/LConn2 -- 11/RConn2
  11-1/RConn3 -- 6/LConn3 -- 13-1/LConn3
  17-1/LConn1 -- 11/RConn1
  12/LConn1 -- load12/LConn1
  31/LConn3 -- T2: 900MVA 20 kV/230 kV3/LConn3
  G2/LConn1 -- Subsystem7/LConn1 -- 31/RConn1 -- Load Flow Bus2/LConn1
  31/LConn2 -- T2: 900MVA 20 kV/230 kV3/LConn2
  12-1/RConn2 -- 7/RConn2
  12-1/RConn3 -- 7/RConn3
  12-1/RConn1 -- 7/RConn1
  11-1/RConn1 -- 6/LConn1 -- 13-1/LConn1
  6-1/RConn2 -- 9-1/RConn2 -- 4/LConn2
  6-1/RConn1 -- 4/LConn1 -- 9-1/RConn1
  3/RConn1 -- load3/LConn1 -- 6-1/LConn1
  3/RConn2 -- load3/LConn2 -- 6-1/LConn2
  6-1/LConn3 -- load3/LConn3 -- 3/RConn3
  23-1/RConn1 -- 14/RConn1 -- 9-1/LConn1
  23-1/RConn2 -- 14/RConn2 -- 9-1/LConn2
  23-1/RConn3 -- 14/RConn3 -- 9-1/LConn3
  6-1/RConn3 -- 4/LConn3 -- 9-1/RConn3
  4/RConn3 -- load4/LConn3 -- 8-1/LConn3
  4/RConn1 -- load4/LConn1 -- 8-1/LConn1
  37-1/LConn3 -- Three-Phase Breaker/LConn3 -- 33/RConn3
  37-1/LConn2 -- Three-Phase Breaker/LConn2 -- 33/RConn2
  37-1/LConn1 -- Three-Phase Breaker/LConn1 -- 33/RConn1
  16/RConn1 -- 25-1/LConn1 -- Subsystem4/LConn1 -- 28-1/RConn1
  25-1/LConn3 -- Subsystem4/LConn3 -- 28-1/RConn3 -- 16/RConn3
  16/RConn2 -- 25-1/LConn2 -- Subsystem4/LConn2 -- 28-1/RConn2
  24-1/LConn3 -- 16/LConn3 -- 26-1/LConn3 -- 27-1/RConn3
  34-1/LConn1 -- Three-Phase Breaker1/LConn1 -- 23/RConn1
  36/LConn3 -- 37-1/RConn3 -- 35-1/RConn3
  36/LConn1 -- 37-1/RConn1 -- 35-1/RConn1
  36/LConn2 -- 37-1/RConn2 -- 35-1/RConn2
  23-1/LConn1 -- Three-Phase Breaker2/RConn1 -- 15/RConn1
  23-1/LConn2 -- Three-Phase Breaker2/RConn2 -- 15/RConn2
  23-1/LConn3 -- Three-Phase Breaker2/RConn3 -- 15/RConn3
  26-1/RConn1 -- T2: 900MVA 20 kV/230 kV10/RConn1 -- 19/LConn1
  26-1/RConn2 -- T2: 900MVA 20 kV/230 kV10/RConn2 -- 19/LConn2
  26-1/RConn3 -- T2: 900MVA 20 kV/230 kV10/RConn3 -- 19/LConn3
  34-1/LConn2 -- Three-Phase Breaker1/LConn2 -- 23/RConn2
  34-1/LConn3 -- Three-Phase Breaker1/LConn3 -- 23/RConn3
  22/RConn2 -- 35-1/LConn2 -- T2: 900MVA 20 kV/230 kV11/RConn2
  T2: 900MVA 20 kV/230 kV11/RConn1 -- 35-1/LConn1 -- 22/RConn1
  22/RConn3 -- 35-1/LConn3 -- T2: 900MVA 20 kV/230 kV11/RConn3
  T2: 900MVA 20 kV/230 kV9/RConn1 -- 20/RConn1
  T2: 900MVA 20 kV/230 kV9/RConn2 -- 20/RConn2
  T2: 900MVA 20 kV/230 kV9/RConn3 -- 20/RConn3
  28-1/LConn1 -- 33/LConn1
  28-1/LConn2 -- 33/LConn2
  28-1/LConn3 -- 33/LConn3
  27-1/LConn1 -- 23/LConn1
  27-1/LConn2 -- 23/LConn2
  T2: 900MVA 20 kV/230 kV12/LConn2 -- 35/LConn2
  35/RConn2 -- G7/LConn2
  T2: 900MVA 20 kV/230 kV12/LConn3 -- 35/LConn3
  35/RConn1 -- Load Flow Bus7/LConn1 -- G7/LConn1
  T2: 900MVA 20 kV/230 kV12/LConn1 -- 35/LConn1
  24-1/RConn1 -- 15/LConn1
  24-1/RConn2 -- 15/LConn2
  24-1/RConn3 -- 15/LConn3
  34/LConn2 -- T2: 900MVA 20 kV/230 kV9/LConn2
  34/LConn3 -- T2: 900MVA 20 kV/230 kV9/LConn3
  G5/LConn3 -- 34/RConn3
  G5/LConn2 -- 34/RConn2
  G5/LConn1 -- 34/RConn1
  27-1/LConn3 -- 23/LConn3
  T2: 900MVA 20 kV/230 kV11/LConn2 -- 24/LConn2
  T2: 900MVA 20 kV/230 kV11/LConn3 -- 24/LConn3
  24/RConn2 -- G6/LConn2
  24/RConn1 -- Load Flow Bus6/LConn1 -- G6/LConn1
  34-1/RConn1 -- 22/LConn1
  34-1/RConn2 -- 22/LConn2
  34-1/RConn3 -- 22/LConn3
  34/LConn1 -- T2: 900MVA 20 kV/230 kV9/LConn1
  24/LConn1 -- T2: 900MVA 20 kV/230 kV11/LConn1
  25/LConn1 -- 39-1/RConn1 -- T2: 900MVA 20 kV/230 kV1/RConn1
  39-1/RConn2 -- 25/LConn2 -- T2: 900MVA 20 kV/230 kV1/RConn2
  T2: 900MVA 20 kV/230 kV1/RConn3 -- 39-1/RConn3 -- 25/LConn3
  1-1/LConn1 -- 2/RConn1 -- 3-1/RConn1
  26/RConn1 -- 41/RConn1 -- 39-1/LConn1
  " 30"/RConn2 -- 17/LConn2 -- 25-1/RConn2
  " 30"/RConn3 -- 17/LConn3 -- 25-1/RConn3
  26/LConn3 -- Subsystem5/LConn3 -- Three-Phase V-I Measurement1/RConn3 -- 42/RConn3
  42/RConn2 -- Subsystem5/LConn2 -- Three-Phase V-I Measurement1/RConn2 -- 26/LConn2
  load27/LConn1 -- 41/LConn1 -- 27/LConn1
  " 30"/RConn1 -- 17/LConn1 -- 25-1/RConn1
  26/RConn3 -- 39-1/LConn3 -- 41/RConn3
  load27/LConn3 -- 41/LConn3 -- 27/LConn3
  28/RConn2 -- 42/LConn2 -- 44/RConn2
  28/RConn1 -- 42/LConn1 -- 44/RConn1
  42/LConn3 -- 44/RConn3 -- 28/RConn3
  30/RConn3 -- T2: 900MVA 20 kV/230 kV2/LConn3
  30/RConn1 -- T2: 900MVA 20 kV/230 kV2/LConn1
  30/RConn2 -- T2: 900MVA 20 kV/230 kV2/LConn2
  30/LConn1 -- Load Flow Bus/LConn1 -- G10/LConn1
  30/LConn2 -- G10/LConn2
  30/LConn3 -- G10/LConn3
  37/RConn2 -- T2: 900MVA 20 kV/230 kV1/LConn2
  37/LConn2 -- G8/LConn2
  37/RConn3 -- T2: 900MVA 20 kV/230 kV1/LConn3
  37/LConn3 -- G8/LConn3
  37/LConn1 -- Load Flow Bus8/LConn1 -- G8/LConn1
  37/RConn1 -- T2: 900MVA 20 kV/230 kV1/LConn1
  29-1/LConn1 -- 17/RConn1
  29-1/LConn2 -- 17/RConn2
  29-1/LConn3 -- 17/RConn3
  27/RConn1 -- " 30"/LConn1
  T2: 900MVA 20 kV/230 kV7/LConn1 -- 38/LConn1
  T2: 900MVA 20 kV/230 kV7/LConn3 -- 38/LConn3
  T2: 900MVA 20 kV/230 kV7/LConn2 -- 38/LConn2
  T2: 900MVA 20 kV/230 kV7/RConn1 -- 29/LConn1
  29/LConn2 -- T2: 900MVA 20 kV/230 kV7/RConn2
  T2: 900MVA 20 kV/230 kV7/RConn3 -- 29/LConn3
  28/LConn1 -- Subsystem8/LConn1
  28/LConn2 -- Subsystem8/LConn2
  28/LConn3 -- Subsystem8/LConn3
  38/RConn3 -- Load Flow Bus9/LConn1 -- G9/LConn3
  38/RConn2 -- G9/LConn2
  38/RConn1 -- G9/LConn1
  1-1/RConn3 -- 1/LConn3
  1-1/RConn2 -- 1/LConn2
  1-1/RConn1 -- 1/LConn1
  26/RConn2 -- 41/RConn2 -- 39-1/LConn2
  " 30"/LConn2 -- 27/RConn2
  " 30"/LConn3 -- 27/RConn3
  8-1/LConn2 -- load4/LConn2 -- 4/RConn2
  T2: 900MVA 20 kV/230 kV4/LConn3 -- 13-1/RConn3 -- 11/LConn3
  12/LConn2 -- load12/LConn2
  12/LConn3 -- load12/LConn3
  T2: 900MVA 20 kV/230 kV8/LConn1 -- 19/RConn1
  T2: 900MVA 20 kV/230 kV8/LConn2 -- 19/RConn2
  T2: 900MVA 20 kV/230 kV8/LConn3 -- 19/RConn3
  T2: 900MVA 20 kV/230 kV8/RConn3 -- 20/LConn3
  T2: 900MVA 20 kV/230 kV8/RConn2 -- 20/LConn2
  T2: 900MVA 20 kV/230 kV8/RConn1 -- 20/LConn1
  43/RConn1 -- Three-Phase V-I Measurement1/LConn1
  43/RConn2 -- Three-Phase V-I Measurement1/LConn2
  43/RConn3 -- Three-Phase V-I Measurement1/LConn3
  load27/LConn2 -- 41/LConn2 -- 27/LConn2
  8-1/RConn3 -- 5/LConn3
  8-1/RConn2 -- 5/LConn2
  8-1/RConn1 -- 5/LConn1
  14-1/LConn3 -- 7/LConn3
  14-1/LConn2 -- 7/LConn2
  14-1/LConn1 -- 7/LConn1
  load8/LConn1 -- 8/RConn1
  8/RConn2 -- load8/LConn2
  load8/LConn3 -- 8/RConn3
  4-1/LConn1 -- 25/RConn1 -- Subsystem2/LConn1
  25/RConn2 -- Subsystem2/LConn2 -- 4-1/LConn2
  4-1/LConn3 -- Subsystem2/LConn3 -- 25/RConn3
  T2: 900MVA 20 kV/230 kV2/RConn3 -- 4-1/RConn3 -- 2/LConn3
  4-1/RConn2 -- 2/LConn2 -- T2: 900MVA 20 kV/230 kV2/RConn2
  4-1/RConn1 -- T2: 900MVA 20 kV/230 kV2/RConn1 -- 2/LConn1
  43/LConn1 -- 44/LConn1 -- Subsystem3/LConn1 -- 29/RConn1
  43/LConn2 -- 44/LConn2 -- Subsystem3/LConn2 -- 29/RConn2
  43/LConn3 -- 44/LConn3 -- Subsystem3/LConn3 -- 29/RConn3
  42/RConn1 -- Subsystem5/LConn1 -- Three-Phase V-I Measurement1/RConn1 -- 26/LConn1
  3/LConn1 -- 3-1/LConn1 -- 7-1/RConn1
  3-1/LConn2 -- 7-1/RConn2 -- 3/LConn2
  3-1/LConn3 -- 7-1/RConn3 -- 3/LConn3
  1-1/LConn2 -- 2/RConn2 -- 3-1/RConn2
  1-1/LConn3 -- 2/RConn3 -- 3-1/RConn3
  7-1/LConn1 -- 29-1/RConn1 -- 18/RConn1
  7-1/LConn2 -- 29-1/RConn2 -- 18/RConn2
  7-1/LConn3 -- 29-1/RConn3 -- 18/RConn3
  10-1/LConn1 -- 11-1/LConn1 -- 5/RConn1
  5/RConn2 -- 11-1/LConn2 -- 10-1/LConn2
  10-1/LConn3 -- 11-1/LConn3 -- 5/RConn3
  6/RConn3 -- T2: 900MVA 20 kV/230 kV3/RConn3 -- 12-1/LConn3 -- load7/LConn3
  T2: 900MVA 20 kV/230 kV4/RConn1 -- T2: 900MVA 20 kV/230 kV5/RConn1 -- 12/RConn1
  T2: 900MVA 20 kV/230 kV4/RConn2 -- T2: 900MVA 20 kV/230 kV5/RConn2 -- 12/RConn2
  T2: 900MVA 20 kV/230 kV4/RConn3 -- T2: 900MVA 20 kV/230 kV5/RConn3 -- 12/RConn3
  14/LConn1 -- 22-1/LConn1
  22-1/LConn2 -- 14/LConn2
  14/LConn3 -- 22-1/LConn3
  24-1/LConn2 -- 26-1/LConn2 -- 27-1/RConn2 -- 16/LConn2
  24-1/LConn1 -- 16/LConn1 -- 27-1/RConn1 -- 26-1/LConn1
  24/RConn3 -- G6/LConn3
  35/RConn3 -- G7/LConn3
  T2: 900MVA 20 kV/230 kV12/RConn1 -- Subsystem1/LConn1 -- 36/RConn1
  T2: 900MVA 20 kV/230 kV12/RConn2 -- 36/RConn2 -- Subsystem1/LConn2
  T2: 900MVA 20 kV/230 kV12/RConn3 -- 36/RConn3 -- Subsystem1/LConn3
  21/LConn2 -- G4/LConn2
  21/LConn1 -- Load Flow Bus4/LConn1 -- G4/LConn1
  21/LConn3 -- G4/LConn3
  T2: 900MVA 20 kV/230 kV10/LConn3 -- 21/RConn3
  T2: 900MVA 20 kV/230 kV10/LConn2 -- 21/RConn2
  T2: 900MVA 20 kV/230 kV10/LConn1 -- 21/RConn1
  T2: 900MVA 20 kV/230 kV3/LConn1 -- 31/LConn1
  Subsystem6/LConn1 -- 18/LConn1
  Subsystem6/LConn2 -- 18/LConn2
  Subsystem6/LConn3 -- 18/LConn3
  Three-Phase Breaker/RConn1 -- load24/LConn1
  load24/LConn2 -- Three-Phase Breaker/RConn2
  Three-Phase Breaker/RConn3 -- load24/LConn3
  load21/LConn1 -- Three-Phase Breaker1/RConn1
  Three-Phase Breaker1/RConn2 -- load21/LConn2
  load21/LConn3 -- Three-Phase Breaker1/RConn3
  Three-Phase Breaker2/LConn1 -- load15/LConn1
  Three-Phase Breaker2/LConn2 -- load15/LConn2
  Three-Phase Breaker2/LConn3 -- load15/LConn3
